simulink model "VTOL_Model_Real"  (R2025b)
settings: Solver=VariableStepAuto  StartTime=0.0  StopTime=10.0  RelTol=1e-3
values from neighbouring files (symbols this model uses):
  C = sysD.C    [Assessment_Code.m]
  student_ID = 11908203    [Assessment_Code.m]
  Ts = 0.01    [Assessment_Code.m]
  x0 = x_bar + [m*(-x_ref); 0; m*(-y_ref); 0; 0; 0]    [Assessment_Code.m]
libraries: simulink x1
settings Model: Creator=froessil  LastModifiedBy=froessil

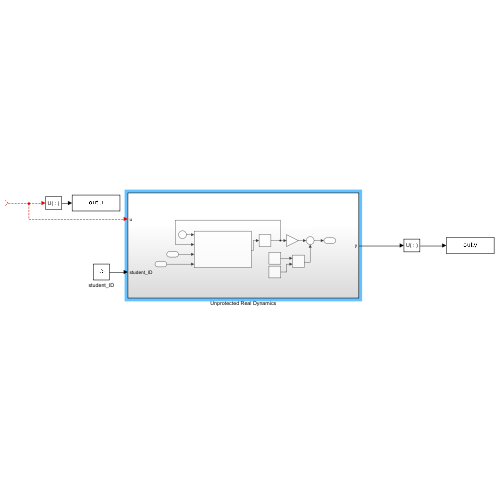
[thumbnail: Simulink's stored preview of the top-level diagram]
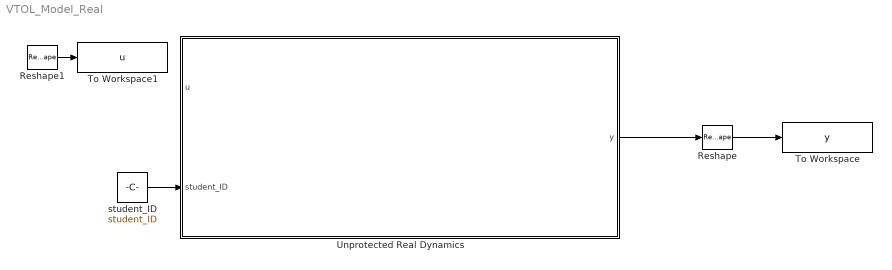
== system VTOL_Model_Real ==
  Reshape : Reshape
  Reshape1 : Reshape
  To Workspace : ToWorkspace  VariableName=y  SampleTime=-1
      settings: Save2DSignal=2-D array (concatenate along first dimension)
  To Workspace1 : ToWorkspace  VariableName=u  SaveFormat=Timeseries  SampleTime=-1
  Unprotected Real Dynamics : Subsystem
  student_ID : Constant  Value=student_ID
  wires:
  Unprotected Real Dynamics/1(y) -> Reshape/1
  student_ID/1 -> Unprotected Real Dynamics/2(student_ID)
  Reshape/1 -> To Workspace/1
  Reshape1/1 -> To Workspace1/1
  ? -> Unprotected Real Dynamics/1(u), Reshape1/1

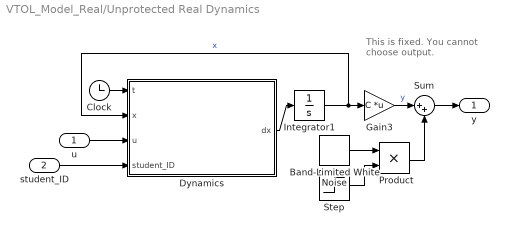
== system VTOL_Model_Real/Unprotected Real Dynamics ==
  note: This is fixed. You cannot choose output.
  u : Inport
  student_ID : Inport  Port=2
  Band-Limited White Noise : simulink/Sources/Band-Limited White Noise  Cov=[0.001]  Ts=Ts  seed=student_ID
  Clock : Clock
  "Dynamics " : MATLAB Function  TreatAsAtomicUnit=on
  Gain3 : Gain  Gain=C  Multiplication=Matrix(K*u)
  Integrator1 : Integrator  InitialCondition=x0
  Product : Product
  Step : Step  Time=0  SampleTime=0
  Sum : Sum  Inputs=|++
  y : Outport
  wires:
  Integrator1/1 -> "Dynamics "/2(x), Gain3/1  "x"
  Clock/1 -> "Dynamics "/1(t)
  u/1 -> "Dynamics "/3(u)
  "Dynamics "/1(dx) -> Integrator1/1
  student_ID/1 -> "Dynamics "/4(student_ID)
  Gain3/1 -> Sum/1  "y"
  Band-Limited White Noise/1 -> Product/1
  Product/1 -> Sum/2
  Step/1 -> Product/2
  Sum/1 -> y/1

== matlab function VTOL_Model_Real/Unprotected Real Dynamics/Dynamics  ==
  data: t input; x input; u input; student_ID input; dx output
function dx = VTOL_Dynamics(t, x, u, student_ID)
dx = zeros(6,1);
dx = VTOL_Dynamics(t, x, u, student_ID);
